simulink model "step3e"  (Simulink 8.5)
settings: Solver=ode23t  SolverMode=SingleTasking  StartTime=0.0  StopTime=0.249  FixedStep=1e-4  RelTol=1e-4  AbsTol=1e-6
undefined symbols (not defined in the file or in its folder): den, dx, num
libraries: powerlib x13, elements x1
settings Model: Creator=PC  LastModifiedBy=PC
settings DataIOCC: LimitDataPoints=off
settings OptimizationCC: BlockReduction=off  BooleanDataType=off  ExpressionDepthLimit=128
settings DebuggingCC: SaveWithParameterizedLinksMsg=none  SignalResolutionControl=TryResolveAllWithWarning  MultiTaskDSMMsg=warning  MultiTaskCondExecSysMsg=none  FcnCallInpInsideContextMsg=EnableAllAsError  StateNameClashWarn=none
settings HardwareCC: TargetUnknown=on
settings RTWCC: TemplateMakefile=grt_vc.tmf

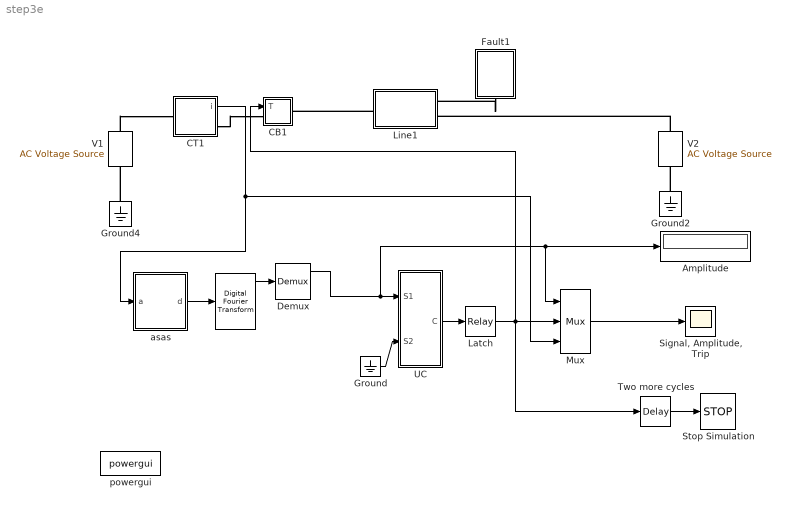
== system step3e ==
  " " : elements/   fo=60  window_size=20  harmonic=[1 2 3 4 5]
  Amplitude : Display
  CB1 : Subsystem  mask(CB){t_op=15}
      mask prompts: t_op "Operating time [ms]"
      mask Display: disp('CB')
  CT1 : Subsystem  mask(CT){Prim=1600, Sec=1}
      mask prompts: Prim "Primary Current [A]"; Sec "Secondary Current [A]"
      mask Display: disp('CT')
  Demux : Demux  Outputs=2
  Fault1 : Subsystem  mask(Fault){RF=0.1, tf=2/60}
      mask prompts: RF "Resistance [ohm]"; tf "Time [sec]"
      mask Display: plot(0,0,100,100,[44,47,56,38,50],[23,8,64,44,97],[56,47],[25,8])
  Ground : Ground
  Ground2 : powerlib/Elements/Ground  LConnTagsString=a
  Ground4 : powerlib/Elements/Ground  LConnTagsString=a
  Latch : Relay  OnSwitchValue=0.9  OffSwitchValue=-2
  Line1 : Subsystem  mask(Simple Line){R=6, X=60, p=0.5}
      mask prompts: R "Resistance [ohm]"; X "Reactance [ohm]"; p "Fault location [pu]"
      mask init:
      | R1=R*p; R2=R*(1-p);
      | L1=X*p/(2*pi*60);L2=X*(1-p)/(2*pi*60);
  Mux : Mux  Inputs=3
  "Signal, Amplitude, Trip" : Scope
      settings: TickLabels=on  YMin=-175  YMax=250
  Stop Simulation : Stop
  Two more cycles : TransportDelay  DelayTime=2/60
  UC : Subsystem  mask(Universal Comparator){type2=Signal-Time, sign=>, Ipickup=0.6, k1=0.95, type1=RI Inverse, type3=Present value, k=0.015, fs=20*60}
      mask prompts: type2 "Type of comparison"; Ipickup "Pick-up value:"; k1 "Ratio of reset to pick-up:"; type1 "Type of Time dependency"; type3 "I-t emulation method"; k "Time parameter (seconds):"; fs "Sampling frecuency (Hz):"
      mask help: This block is an Universal Comparator. It can perform a comparison between a signal an a threshold or two signals. It can also emulate some time-signal characteristics.
      mask init:
      | switch type2,
      |    case 1,
      |        %signal-threshold
      |        if sign ==1
      |           %S1>S2
      |           aux=0;
      |        else
      |           %S1<S2
      |           aux=1;
      |        end;
      |    case 2,
      |        %Signal-Signal
      |       if sign ==1
      |           aux=2;
      |    	else
      |          aux=3;
      |       end;
      |    case 3,
      |       %signal-time
      |       if type3==1
      |          %instantaneous value of input signal
      |          switch type1,
      |             case 1,
      |                %time defined
      |                aux=4;
      |             case 2,
      |                %inverse time
      |                aux=6;
      |             case 3,
      |                %very inverse
      |                aux=7;
      |             case 4,
      |                %extremely inverse
      |                aux=8;
      |             case 5,
      |                %RI inverse
      |                aux=9;
      |             case 6,
      |                %Long time inverse
      |                aux=10;
      |             otherwise,
      |                aux=0;
      |          end;
      |       else
      |          switch type1,
      |             case 1,
      |                %time defined
      |                aux=5;
      |             case 2,
      |                %inverse time
      |                aux=11;
      |             case 3,
      |                %very inverse
      |                aux=12;
      |             case 4,
      |                %extremely inverse
      |                aux=13;
      |             case 5,
      |                %RI inverse
      |                aux=14;
      |             case 6,
      |                %Long time inverse
      |                aux=15;
      |             otherwise,
      |                aux=0;
      |          end;
      |       end;
      |    otherwise,
      |          aux=0;
      | end;
      mask TypeOptions type2: Signal-Threshold | Signal-Signal | Signal-Time
      mask TypeOptions sign: > | <
      mask TypeOptions type1: Time defined | Standard Inverse | Very Inverse | Extra Inverse | RI Inverse | Long Time Inverse
      mask TypeOptions type3: Present value | integration
      mask Display: disp('UC');
  V1 : powerlib/Electrical Sources/AC Voltage Source  Amplitude=100  Phase=0  Frequency=60  SampleTime=0  Measurements=None
  V2 : powerlib/Electrical Sources/AC Voltage Source  Amplitude=100  Phase=170  Frequency=60  SampleTime=0  Measurements=None
  "asas  " : Subsystem  mask(Data Adquisition Board){filter=off, approx=Butterworth, order=3, numerator=[], denominator=[], freq=180, resdis=off, vertres=16, xmax=10, winsize=20, G=1.0, fs=60*20}
      mask prompts: filter "Disable Analog Filter"; approx "Filter approximation"; numerator "Free expression filter: numerator(descending order of s)"; denominator "Free expression filter: denominator:"; freq "Cut-off frequency"; resdis "Disable Vertical Resolution"; vertres "Vertical Resolution: No. of bits"; xmax "Vertical Resolution: signal range"; winsize "Window size"; G "Gain"; fs "Sampling frequency"
      mask help: Takes the instantaneous value of the input signal and convert it to the data window of samples.
      mask init:
      | dab1
      mask TypeOptions approx: Bessel | Tschebyscheff | Butterworth | free expression
      mask TypeOptions order: 2 | 3 | 4
      mask TypeOptions vertres: 8 | 12 | 16
      mask Display: disp('DAB')
  powergui : powerlib/powergui  SimulationMode=Continuous  SolverType=Tustin/Backward Euler (TBE)  SampleTime=0  frequency=60  SPID=off  DisableSnubberDevices=off  DisableRonSwitches=off  DisableVfSwitches=off  SwTol=0  DisplayEquations=off  Interpol=off  methode=off  Ts=0  FunctionMessages=off  echomessages=off  HookPort=off  EnableUseOfTLC=off  x0status=blocks  frequencyindice=60  Pbase=100e6  ErrMax=1e-4  Iterations=50  UnitsV=kV  UnitsW=MW  buscounter=0  RestoreLinks=warning  ResistiveCurrentMeasurement=off  Frange=[0:2:500]  Ylog=off  Xlog=on  ShowGrid=off  save=off  variable=ZData  structure=0  ZoomFFT=on  StartTime=0.0  cycles=1  DisplayStyle=1  fundamental=60  FreqAxis=off  MaxFrequency=1000  frequencyindicesteady=1  RmsSteady=1  display=off
  wires:
  Latch/1 -> CB1/1(T), Two more cycles/1, Mux/2
  UC/1(C) -> Latch/1
  Two more cycles/1 -> Stop Simulation/1
  Mux/1 -> "Signal, Amplitude, Trip"/1
  Ground/1 -> UC/2(S2)
  "asas  "/1(d) -> " "/1
  " "/1 -> Demux/1
  Demux/1 -> Mux/1, Amplitude/1, UC/1(S1)
  CT1/1(i) -> "asas  "/1(a), Mux/3
  connections:
  CT1/RConn1 -- CB1/LConn1
  V1/RConn1 -- CT1/LConn1
  Ground4/LConn1 -- V1/LConn1
  Line1/LConn1 -- CB1/RConn1
  V2/RConn1 -- Line1/RConn2
  Ground2/LConn1 -- V2/LConn1
  Fault1/LConn1 -- Line1/RConn1

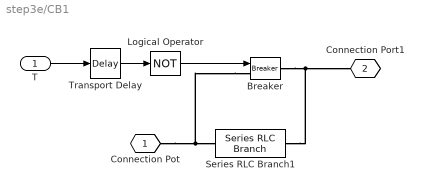
== system step3e/CB1 ==
  T : Inport
  Breaker : powerlib/Elements/Breaker  Tag=PoWeRsYsTeMbLoCk  InitialState=0  SwitchingTimes="[ 1/60  5/60 ]"  External=on  BreakerResistance=0.01  SnubberResistance=1e6  SnubberCapacitance=inf  Measurements=None  MoreParameters=off  NoBreakLoop=off
  Logical Operator : Logic  Operator=NOT  Inputs=1
  Series RLC Branch1 : powerlib/Elements/Series RLC Branch  LConnTagsString=__new0  RConnTagsString=__new0  BranchType=RLC  Resistance=1  Inductance=1e-3  SetiL0=off  InitialCurrent=0  Capacitance=1e-6  Setx0=off  InitialVoltage=0  Measurements=None
  Transport Delay : TransportDelay  DelayTime=t_op/1000
  Connection Pot : PMIOPort  Tag=PMCPort  Port=1  Side=Left
  Connection Port1 : PMIOPort  Tag=PMCPort  Port=2  Side=Right
  wires:
  Logical Operator/1 -> Breaker/1
  Transport Delay/1 -> Logical Operator/1
  T/1 -> Transport Delay/1
  connections:
  Series RLC Branch1/RConn1 -- Connection Port1/RConn1 -- Breaker/RConn1
  Breaker/LConn1 -- Series RLC Branch1/LConn1 -- Connection Pot/RConn1

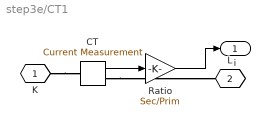
== system step3e/CT1 ==
  CT : powerlib/Measurements/Current Measurement  PhasorSimulation=off  OutputType=Complex  PSBequivalent=0
  Ratio : Gain  Gain=Sec/Prim  SaturateOnIntegerOverflow=on  OutDataTypeStr=Inherit: Same as input  ParamDataTypeStr=Inherit: Same as input
  K : PMIOPort  Tag=PMCPort  Port=1  Side=Left
  L : PMIOPort  Tag=PMCPort  Port=2  Side=Right
  i : Outport  InitialOutput=0
  wires:
  Ratio/1 -> i/1
  CT/1 -> Ratio/1
  connections:
  CT/RConn1 -- L/RConn1
  K/RConn1 -- CT/LConn1

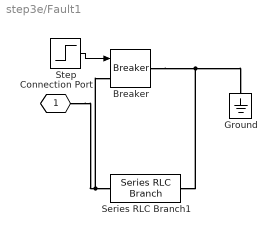
== system step3e/Fault1 ==
  Breaker : powerlib/Elements/Breaker  Tag=PoWeRsYsTeMbLoCk  InitialState=0  SwitchingTimes="[ 1/60  5/60 ]"  External=on  BreakerResistance=0.01  SnubberResistance=1e6  SnubberCapacitance=inf  Measurements=None  MoreParameters=off  NoBreakLoop=off
  Ground : powerlib/Elements/Ground  LConnTagsString=a
  Series RLC Branch1 : powerlib/Elements/Series RLC Branch  LConnTagsString=__new0  RConnTagsString=__new0  BranchType=RLC  Resistance=1  Inductance=1e-3  SetiL0=off  InitialCurrent=0  Capacitance=1e-6  Setx0=off  InitialVoltage=0  Measurements=None
  Step : Step  Time=tf
  Connection Port : PMIOPort  Tag=PMCPort  Port=1  Side=Left
  wires:
  Step/1 -> Breaker/1
  connections:
  Series RLC Branch1/LConn1 -- Breaker/LConn1 -- Connection Port/RConn1
  Series RLC Branch1/RConn1 -- Ground/LConn1 -- Breaker/RConn1

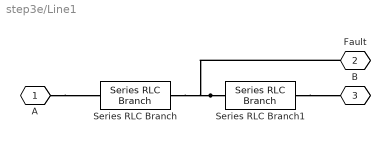
== system step3e/Line1 ==
  Series RLC Branch : powerlib/Elements/Series RLC Branch  LConnTagsString=__new0  RConnTagsString=__new0  BranchType=RL  Resistance=R1  Inductance=L1  SetiL0=off  InitialCurrent=0  Capacitance=1.0  Setx0=off  InitialVoltage=0  Measurements=None
  Series RLC Branch1 : powerlib/Elements/Series RLC Branch  LConnTagsString=__new0  RConnTagsString=__new0  BranchType=RL  Resistance=R2  Inductance=L2  SetiL0=off  InitialCurrent=0  Capacitance=1.0  Setx0=off  InitialVoltage=0  Measurements=None
  A : PMIOPort  Tag=PMCPort  Port=1  Side=Left
  Fault : PMIOPort  Tag=PMCPort  Port=2  Side=Right
  B : PMIOPort  Tag=PMCPort  Port=3  Side=Right
  connections:
  Series RLC Branch1/RConn1 -- B/RConn1
  Series RLC Branch1/LConn1 -- Series RLC Branch/RConn1 -- Fault/RConn1
  A/RConn1 -- Series RLC Branch/LConn1

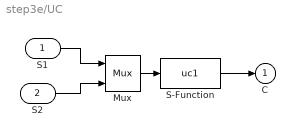
== system step3e/UC ==
  S1 : Inport
  S2 : Inport  Port=2
  Mux : Mux  Inputs=2
  S-Function : S-Function  FunctionName=uc1  Parameters=k,k1,aux,Ipickup,fs
  C : Outport  InitialOutput=0
  wires:
  S-Function/1 -> C/1
  Mux/1 -> S-Function/1
  S1/1 -> Mux/1
  S2/1 -> Mux/2

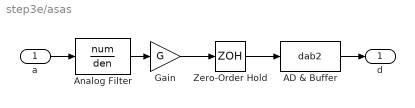
== system step3e/asas   ==
  a : Inport
  AD & Buffer : S-Function  FunctionName=dab2  Parameters=winsize,fs,dx,resdis
  Analog Filter : TransferFcn  Numerator=num  Denominator=den
  Gain : Gain  Gain=G  SaturateOnIntegerOverflow=on  OutDataTypeStr=Inherit: Same as input  ParamDataTypeStr=Inherit: Same as input
  Zero-Order Hold : ZeroOrderHold  SampleTime=1/fs
  d : Outport  InitialOutput=[zeros(winsize,1)]
  wires:
  AD & Buffer/1 -> d/1
  a/1 -> Analog Filter/1
  Zero-Order Hold/1 -> AD & Buffer/1
  Gain/1 -> Zero-Order Hold/1
  Analog Filter/1 -> Gain/1
